simulink model "TP2"  (R2018a)
settings: Solver=VariableStepAuto  StartTime=0.0  StopTime=100  RelTol=1e-3
values from neighbouring files (symbols this model uses):
  A = [0          , 1, 0                 , 0 ... (first row only)    [Valeurs.m]
  B = [0; 0; 0; 1 / J]    [Valeurs.m]
  C = [1, 0, 0, 0 ... (first row only)    [Valeurs.m]
  g = 9.81    [Valeurs.m]
  init = [0.1; 0; 0; 0]    [Valeurs.m]
  J = 0.02    [Valeurs.m]
  L = place( A', C', P_L )'    [Valeurs.m]
  m = 0.6    [Valeurs.m]
  sigma = 0.8    [Valeurs.m]
undefined symbols (not defined in the file or in its folder): K
settings Model: Creator=hbast  LastModifiedBy=hbast

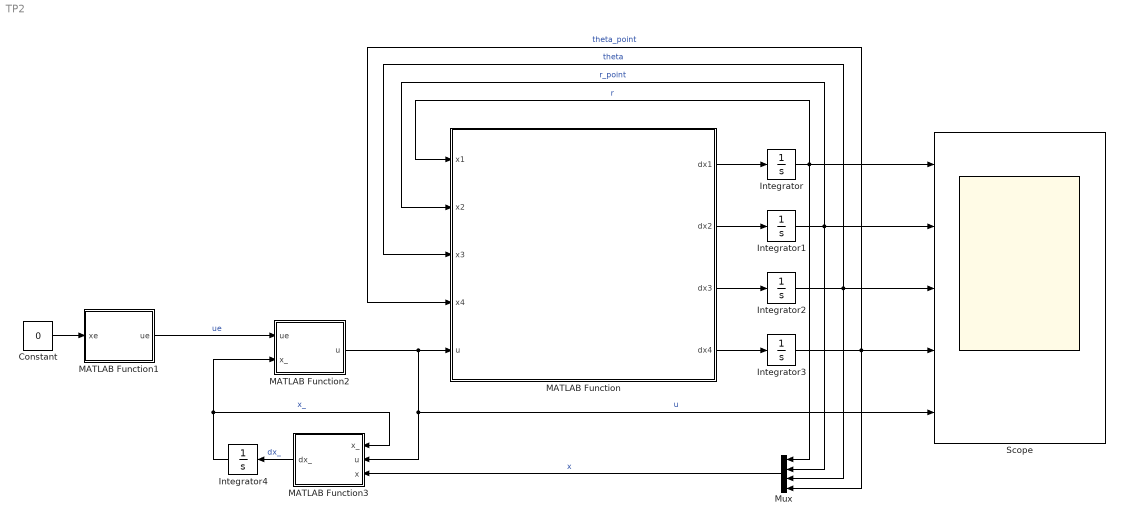
== system TP2 ==
  Constant : Constant  Value=0
  Integrator : Integrator  InitialCondition=init(1)
  Integrator1 : Integrator  InitialCondition=init(2)
  Integrator2 : Integrator  InitialCondition=init(3)
  Integrator3 : Integrator  InitialCondition=init(4)
  Integrator4 : Integrator
  MATLAB Function : MATLAB Function  TreatAsAtomicUnit=on
  MATLAB Function1 : MATLAB Function  TreatAsAtomicUnit=on
  MATLAB Function2 : MATLAB Function  TreatAsAtomicUnit=on
  MATLAB Function3 : MATLAB Function  TreatAsAtomicUnit=on
  Mux : Mux
  Scope : Scope  NumInputPorts=5
  wires:
  MATLAB Function/4(dx4) -> Integrator3/1
  MATLAB Function/3(dx3) -> Integrator2/1
  MATLAB Function/2(dx2) -> Integrator1/1
  MATLAB Function/1(dx1) -> Integrator/1
  Integrator2/1 -> Mux/3, MATLAB Function/3(x3), Scope/3  "theta"
  Integrator3/1 -> Scope/4, MATLAB Function/4(x4), Mux/4  "theta_point"
  Integrator1/1 -> Mux/2, MATLAB Function/2(x2), Scope/2  "r_point"
  Integrator/1 -> Mux/1, MATLAB Function/1(x1), Scope/1  "r"
  MATLAB Function1/1(ue) -> MATLAB Function2/1(ue)  "ue"
  MATLAB Function2/1(u) -> Scope/5, MATLAB Function3/2(u), MATLAB Function/5(u)  "u"
  Integrator4/1 -> MATLAB Function3/1(x_), MATLAB Function2/2(x_)  "x_"
  Mux/1 -> MATLAB Function3/3(x)  "x"
  MATLAB Function3/1(dx_) -> Integrator4/1  "dx_"
  Constant/1 -> MATLAB Function1/1(xe)

== matlab function TP2/MATLAB Function1 ==
  data: xe input; ue output; m parameter; g parameter
function ue = equilibre(xe, m, g)
ue = m * g * xe;
end

== matlab function TP2/MATLAB Function ==
  data: x1 input; x2 input; x3 input; x4 input; u input; dx1 output; dx2 output; dx3 output; dx4 output; J parameter; m parameter; sigma parameter; g parameter
function [dx1, dx2, dx3, dx4] = systeme(x1, x2, x3, x4, u, J, m, sigma, g)
dx1 = x2;
dx2 = ( x1 * x4^2 - g * sin( x3 ) ) / ( 1 + sigma );
dx3 = x4;
dx4 = ( u - m * g * x1 * cos( x3 ) - 2 * m * x1 * x2 * x4 ) / ( J + m * x1^2 );
end

== matlab function TP2/MATLAB Function2 ==
  data: u output; ue input; x_ input; init parameter; K parameter
function u = commande(ue, x_, init, K)
u = ue + K * ( init - x_ );
end

== matlab function TP2/MATLAB Function3 ==
  data: x_ input; u input; dx_ output size=4; x input; A parameter; B parameter; L parameter; C parameter
function dx_ = observateur(x_, u, x, A, B, L, C)
dx_ = A * x_ + B * u + L * C * ( x - x_ );
end
